simulink model "part3"  (R2014a)
settings: Solver=ode45  StartTime=0.0  StopTime=30.0  RelTol=1e-3
libraries: simulink x2
settings Model: Creator=SuperUser  LastModifiedBy=SuperUser

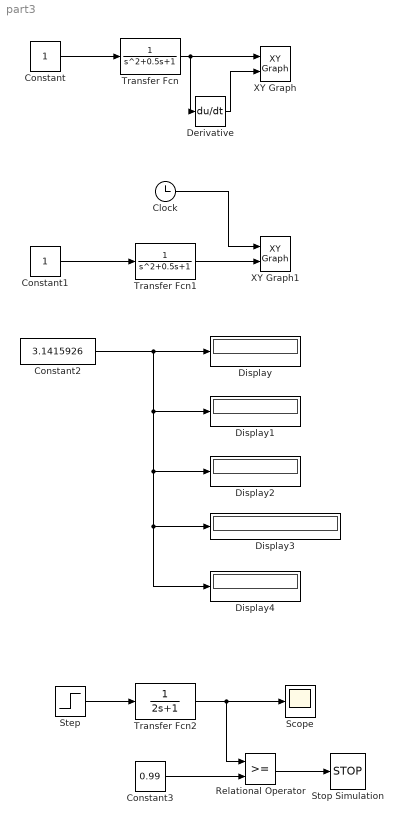
== system part3 ==
  Clock : Clock
      settings: Decimation=30
  Constant : Constant
  Constant1 : Constant
  Constant2 : Constant  Value=3.1415926
  Constant3 : Constant  Value=0.99
  Derivative : Derivative
  Display{,1..4} (5 alike) : Display
      Display2 settings: Format=short_e
      Display3 settings: Format=long_e
  Relational Operator : RelationalOperator  OutDataTypeStr=boolean
  Scope : Scope
  Step : Step  SampleTime=0
  Stop Simulation : Stop
  Transfer Fcn : TransferFcn  Denominator=[1 0.5 1]
  Transfer Fcn1 : TransferFcn  Denominator=[1 0.5 1]
  Transfer Fcn2 : TransferFcn  Denominator=[2 1]
  XY Graph : simulink/Sinks/XY Graph  xmin=0  xmax=2  ymin=-1  ymax=1  st=-1
  XY Graph1 : simulink/Sinks/XY Graph  xmin=0  xmax=30  ymin=0  ymax=2  st=-1
  wires:
  Constant/1 -> Transfer Fcn/1
  Derivative/1 -> XY Graph/2
  Transfer Fcn/1 -> Derivative/1, XY Graph/1
  Constant1/1 -> Transfer Fcn1/1
  Transfer Fcn1/1 -> XY Graph1/2
  Clock/1 -> XY Graph1/1
  Constant2/1 -> Display/1, Display1/1, Display3/1, Display4/1, Display2/1
  Step/1 -> Transfer Fcn2/1
  Transfer Fcn2/1 -> Relational Operator/1, Scope/1
  Constant3/1 -> Relational Operator/2
  Relational Operator/1 -> Stop Simulation/1
